simulink model "step_2nd_system_R2022a"  (R2022a)
settings: Solver=ode4  StartTime=0.0  StopTime=inf  FixedStep=0.001  RelTol=1e-3
settings Model: PacingRate=5  Creator=kawata  LastModifiedBy=kawata
settings ModelReferenceCC: EnableRefExpFcnMdlSchedulingChecks=off
settings RTWCC: Description=Generic Real-Time Target

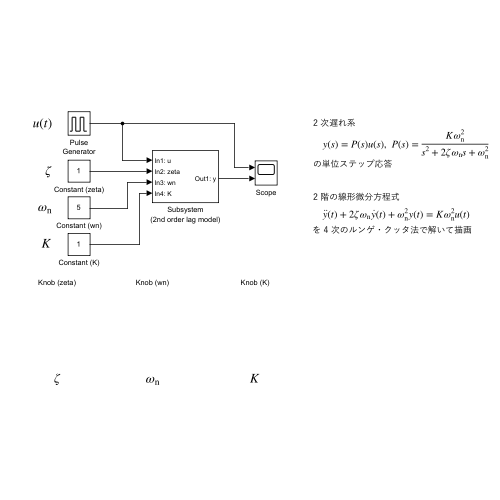
[thumbnail: Simulink's stored preview of the top-level diagram]
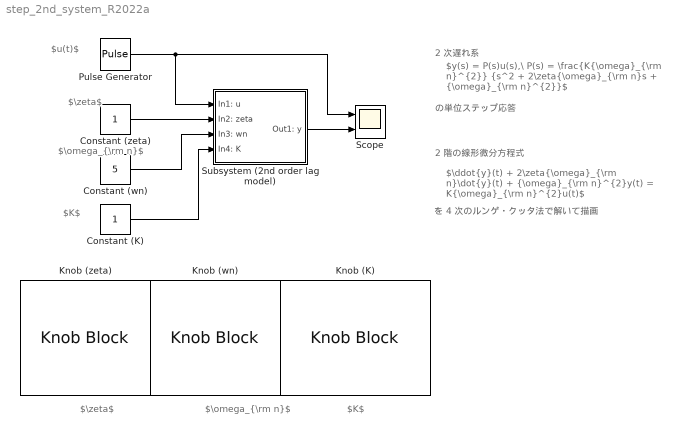
== system step_2nd_system_R2022a ==
  note: 2 次遅れ系
  note: $\omega_{\rm n}$
  note: $\zeta$
  note: $y(s) = P(s)u(s),\ P(s) = \frac{K{\omega}_{\rm n}^{2}} {s^2 + 2\zeta{\omega}_{\rm n}s + {\omega}_{\rm n}^{2}}$
  note: $\zeta$
  note: $\omega_{\rm n}$
  note: $\ddot{y}(t) + 2\zeta{\omega}_{\rm n}\dot{y}(t) + {\omega}_{\rm n}^{2}y(t) = K{\omega}_{\rm n}^{2}u(t)$
  note: の単位ステップ応答
  note: 2 階の線形微分方程式
  note: を 4 次のルンゲ・クッタ法で解いて描画
  note: $K$
  note: $K$
  note: $u(t)$
  Constant (K) : Constant
  Constant (wn) : Constant  Value=5
  Constant (zeta) : Constant
  Knob (K) : KnobBlock  LabelPosition=Hide  ScaleMax=2  TickInterval=0.2
  Knob (wn) : KnobBlock  LabelPosition=Hide  ScaleMax=10
  Knob (zeta) : KnobBlock  LabelPosition=Hide  ScaleMax=2  TickInterval=0.2
  Pulse Generator : DiscretePulseGenerator  PulseType=Time based  Period=10  PulseWidth=50  PhaseDelay=2.5
  Scope : Scope  NumInputPorts=2
  Subsystem (2nd order lag model) : Subsystem
  wires:
  Constant (wn)/1 -> Subsystem (2nd order lag model)/3(In3: wn)
  Constant (zeta)/1 -> Subsystem (2nd order lag model)/2(In2: zeta)
  Pulse Generator/1 -> Subsystem (2nd order lag model)/1(In1: u), Scope/1
  Subsystem (2nd order lag model)/1(Out1: y) -> Scope/2
  Constant (K)/1 -> Subsystem (2nd order lag model)/4(In4: K)

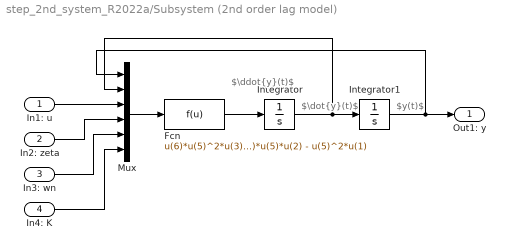
== system step_2nd_system_R2022a/Subsystem (2nd order lag model) ==
  note: $\ddot{y}(t)$
  note: $\dot{y}(t)$
  note: $y(t)$
  In1: u : Inport
  In2: zeta : Inport  Port=2
  In3: wn : Inport  Port=3
  In4: K : Inport  Port=4
  Fcn : Fcn  Expr=u(6)*u(5)^2*u(3) - 2*u(4)*u(5)*u(2) - u(5)^2*u(1)
  Integrator : Integrator
  Integrator1 : Integrator
  Mux : Mux  Inputs=6
  Out1: y : Outport
  wires:
  Integrator/1 -> Mux/2, Integrator1/1
  Mux/1 -> Fcn/1
  In2: zeta/1 -> Mux/4
  In1: u/1 -> Mux/3
  In3: wn/1 -> Mux/5
  Integrator1/1 -> Out1: y/1, Mux/1
  Fcn/1 -> Integrator/1
  In4: K/1 -> Mux/6
